simulink model "Headway_control"  (R2021a)
settings: Solver=VariableStepAuto  StartTime=0.0  StopTime=600  RelTol=1e-3
values from neighbouring files (symbols this model uses):
  Kd = 132.1324    [Headway_Controller_Design.m]
  Ki = 0.093505    [Headway_Controller_Design.m]
  Kp = 8.4948    [Headway_Controller_Design.m]
  plant_den = [1 1/50.5355]    [Headway_Controller_Design.m]
  plant_num = 9.22123*1e-4    (= 0.000922123)    [Headway_Controller_Design.m]
libraries: pid_lib x1, simulink x1
settings Model: Creator=ChOm1  LastModifiedBy=User
settings SolverCC: AlgebraicLoopSolver=TrustRegion
settings DebuggingCC: SFMachineParentedDataDiag=warning

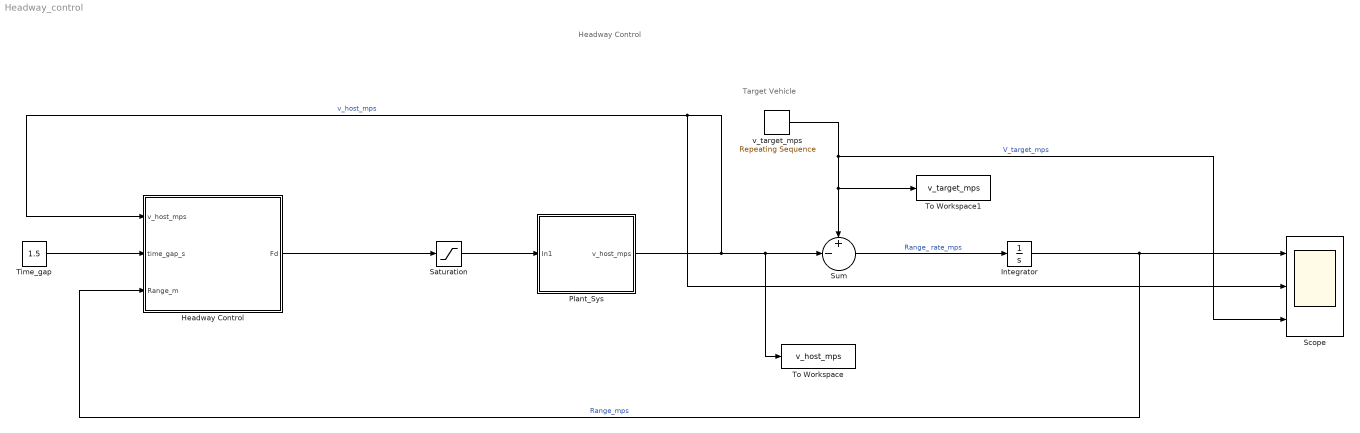
== system Headway_control ==
  note: Headway Control
  note: Target Vehicle
  Headway Control : Subsystem
  Integrator : Integrator
  Plant_Sys : Subsystem
  Saturation : Saturate  UpperLimit=1000  LowerLimit=-1000
  Scope : Scope  NumInputPorts=3
  Sum : Sum  Inputs=+-|
  Time_gap : Constant  Value=1.5
  To Workspace : ToWorkspace  VariableName=v_host_mps  SaveFormat=Timeseries  SampleTime=-1
  To Workspace1 : ToWorkspace  VariableName=v_target_mps  SaveFormat=Timeseries  SampleTime=-1
  v_target_mps : simulink/Sources/Repeating Sequence  rep_seq_t=[0 150 250 350 600]  rep_seq_y=[32 22 22 28 28]
  wires:
  Headway Control/1(Fd) -> Saturation/1
  Plant_Sys/1(v_host_mps) -> To Workspace/1, Sum/2, Headway Control/1(v_host_mps), Scope/2  "v_host_mps"
  v_target_mps/1 -> To Workspace1/1, Sum/1, Scope/3  "V_target_mps"
  Sum/1 -> Integrator/1  "Range_ rate_mps"
  Integrator/1 -> Headway Control/3(Range_m), Scope/1  "Range_mps"
  Time_gap/1 -> Headway Control/2(time_gap_s)
  Saturation/1 -> Plant_Sys/1(In1)

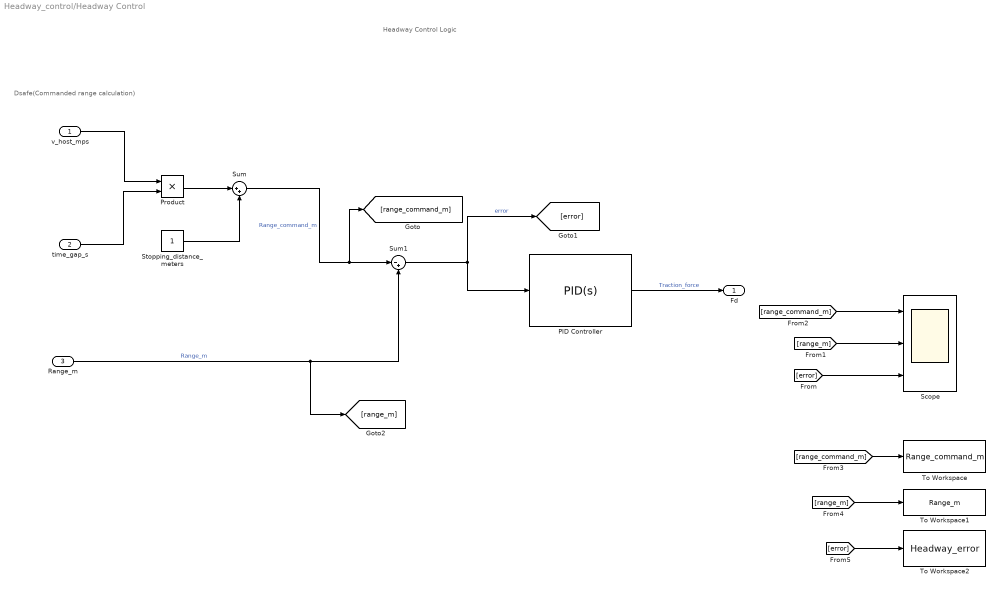
== system Headway_control/Headway Control ==
  note: Headway Control Logic
  note: Dsafe(Commanded range calculation)
  v_host_mps : Inport
  time_gap_s : Inport  Port=2
  Range_m : Inport  Port=3
  PID Controller : pid_lib/PID Controller  Controller=PID  Form=Parallel  TimeDomain=Continuous-time  UseExternalTs=off  SampleTime=-1  IntegratorMethod=Forward Euler  FilterMethod=Forward Euler  ControllerParametersSource=internal  P=Kp  I=Ki  D=Kd  UseFilter=on  N=0.812411488539453  TunerSelectOption=Transfer Function Based (PID Tuner App)  InitialConditionSource=internal  InitialConditionForIntegrator=0  InitialConditionForFilter=0  DifferentiatorICPrevScaledInput=0  ExternalReset=none  TrackingMode=off  Kt=1  LimitOutput=off  SatLimitsSource=internal  UpperSaturationLimit=inf  LowerSaturationLimit=-inf  LinearizeAsGain=on  AntiWindupMode=none  Kb=1  POutMin=[]  POutMax=[]  IOutMin=[]  IOutMax=[]  DOutMin=[]  DOutMax=[]  NOutMin=[]  NOutMax=[]  SumOutMin=[]  SumOutMax=[]  SaturationOutMin=[]  SaturationOutMax=[]  PParamMin=[]  PParamMax=[]  IParamMin=[]  IParamMax=[]  DParamMin=[]  DParamMax=[]  NParamMin=[]  NParamMax=[]  KbParamMin=[]  KbParamMax=[]  KtParamMin=[]  KtParamMax=[]  KbOutMin=[]  KbOutMax=[]  KtOutMin=[]  KtOutMax=[]  IntegratorOutMin=[]  IntegratorOutMax=[]  FilterOutMin=[]  FilterOutMax=[]  SumI1OutMin=[]  SumI1OutMax=[]  SumI2OutMin=[]  SumI2OutMax=[]  SumI3OutMin=[]  SumI3OutMax=[]  SumI4OutMin=[]  SumI4OutMax=[]  SumDOutMin=[]  SumDOutMax=[]  DifferentiatorOutMin=[]  DifferentiatorOutMax=[]  FilterDiffOutCoefMin=[]  FilterDiffOutCoefMax=[]  ReciprocalOutMin=[]  ReciprocalOutMax=[]  SumDenOutMin=[]  SumDenOutMax=[]  SumNumOutMin=[]  SumNumOutMax=[]  DivideOutMin=[]  DivideOutMax=[]  UdiffTsProdOutMin=[]  UdiffTsProdOutMax=[]  NTsProdOutMin=[]  NTsProdOutMax=[]  UintegralTsProdOutMin=[]  UintegralTsProdOutMax=[]  UngainTsProdOutMin=[]  UngainTsProdOutMax=[]  IntegratorContinuousStateAttributes=''  IntegratorStateMustResolveToSignalObject=off  IntegratorRTWStateStorageClass=Auto  FilterContinuousStateAttributes=''  FilterStateMustResolveToSignalObject=off  FilterRTWStateStorageClass=Auto  ParallelPVariant=InternalParameters  IdealPVariant=Disabled  IVariant=InternalParameters  DVariant=InternalParameters  IntegratorVariant=Continuous  SatVariant=Disabled  AWVariant=Passthrough  PCopyVariant=Disabled  TRVariant=Disabled  FdbkBlocksVariant=Forward  IdealPFdbkVariant=Disabled  SatFdbkVariant=Disabled  DerivativeFilterVariant=ContFilter  NVariant=InternalParameters  NCopyVariant=Disabled  FilterICVariant=InternalICsFilter  IntegratorICVariant=InternalICs  ExternalResetVariant=Disabled  TRSumVariant=Passthrough  SumFdbkVariant=Disabled  SumVariant=Sum_PID  TsampFilterVariant=InternalTs  TsampNgainVariant=Passthrough  TsampIntegralVariant=Passthrough  ExternalSaturationOutDataTypeStr=Inherit: Same as second input
  Product : Product
  Scope : Scope  NumInputPorts=3
  Stopping_distance_meters : Constant
  Sum : Sum  Inputs=|++
  Sum1 : Sum  Inputs=|-+
  To Workspace : ToWorkspace  VariableName=Range_command_m  SampleTime=-1
  To Workspace1 : ToWorkspace  VariableName=Range_m  SampleTime=-1
  To Workspace2 : ToWorkspace  VariableName=Headway_error  SaveFormat=Timeseries  SampleTime=-1
  Fd : Outport
  wires:
  v_host_mps/1 -> Product/1
  time_gap_s/1 -> Product/2
  Stopping_distance_meters/1 -> Sum/2
  Product/1 -> Sum/1
  Sum/1 -> [range_command_m], Sum1/1  "Range_command_m"
  Range_m/1 -> [range_m], Sum1/2  "Range_m"
  Sum1/1 -> [error], PID Controller/1  "error"
  PID Controller/1 -> Fd/1  "Traction_force"
  [error] -> Scope/3
  [range_m] -> Scope/2
  [range_command_m] -> Scope/1
  [range_command_m] -> To Workspace/1
  [range_m] -> To Workspace1/1
  [error] -> To Workspace2/1

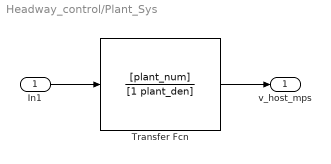
== system Headway_control/Plant_Sys ==
  In1 : Inport
  Transfer Fcn : TransferFcn  Numerator=[plant_num]  Denominator=[1 plant_den]
  v_host_mps : Outport
  wires:
  In1/1 -> Transfer Fcn/1
  Transfer Fcn/1 -> v_host_mps/1
